simulink model "ThreeLevel_Ttype_OffGrid_Inverter_Sim"  (R2022b)
settings: Solver=FixedStepAuto  StartTime=0.0  StopTime=1  FixedStep=1e-6  RelTol=1e-3
undefined symbols (not defined in the file): L1
libraries: spsSeriesRLCBranchLib x14, spsMosfetLib x12, spsRMSLib x10, slpidlib x5, simulink x3, spsThreePhaseVIMeasurementLib x3, spsVoltageMeasurementLib x3, spsDCVoltageSourceLib x1, spsGroundLib x1, spsPower3phInstantaneousLib x1, sps_lib x1
(part 1 of 2)
settings Model: Creator=XIAO  LastModifiedBy=XIAO
settings SolverCC: AutoInsertRateTranBlk=on
settings DataIOCC: ReturnWorkspaceOutputs=off

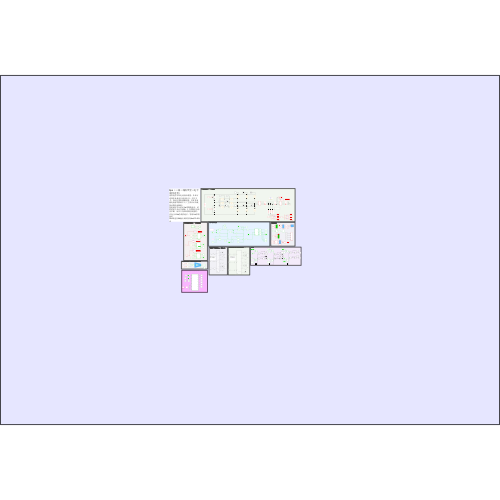
[thumbnail: Simulink's stored preview of the top-level diagram]
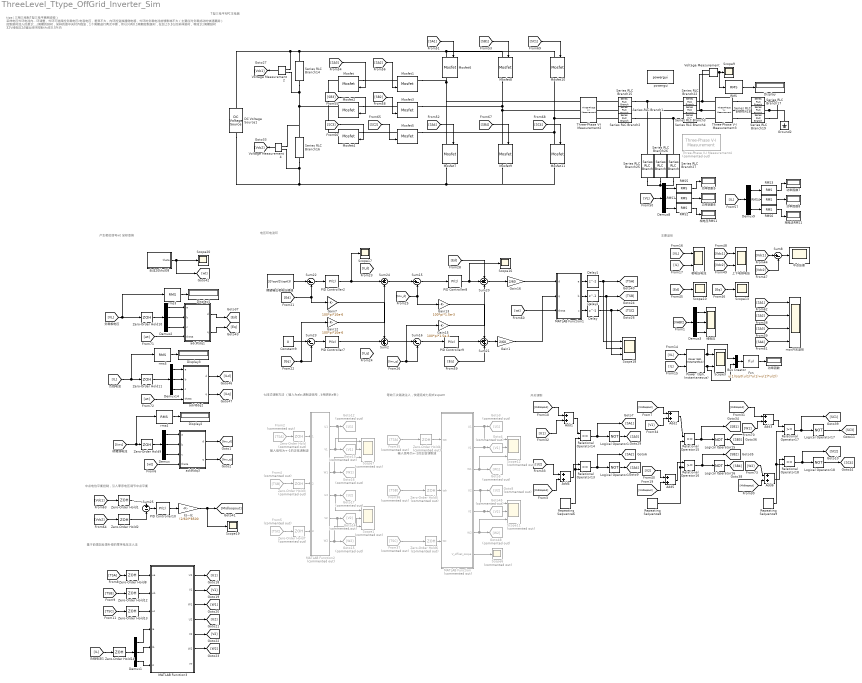
== system ThreeLevel_Ttype_OffGrid_Inverter_Sim ==
  note: 基于前馈加反馈补偿的零序电压注入法
  note: tips（三相三线制T型三电平离网逆变）
      | 采样电压外环电流内环调整，外环可选择控负载电压/电容电压，差异不大，内环控变换器侧电感，外环的负载电流前馈影响不大（主要应对负载扰动的快速跟踪）
      | 控制延时加入的是1ts周期的延时，采样的是中央对齐载波，1个周期进行两次中断，所以只有0.5周期控制延时，在加上0.5ts的采样延时，等效1ts周期延时
      | 32V线电压2A输出闭环控制thd在0.5%内
  note: T型三电平NPC主电路
  note: 主要波形
  note: 产生相位信号wt 坐标变换
  note: 电压环电流环
  note: 中点电位平衡控制，引入零序电压调节中点平衡
  note: 开关调制
  note: 输入信号为+-1的正弦调制波
  note: 等效三次谐波注入，快速完成七段式svpwm
  note: 七段式调制方法
      | （输入为abc调制波信号，b相滞后a相）
  note: 输入信号为+-1的正弦调制波
  Add{1..6} (6 alike) : Sum
  Bus Creator : BusCreator  Inputs=2
  Constant9 : Constant  Value=0
  DC Voltage Source1 : spsDCVoltageSourceLib/DC Voltage Source  Amplitude=60  Measurements=None
  Delay : Delay  DelayLength=1
  Delay1 : Delay  DelayLength=1
  Delay2 : Delay  DelayLength=1
  Demux{,1..3,8..9,14} (7 alike) : Demux  Outputs=3
  Display{,1..3} (4 alike) : Display
  Fcn : Fcn  Expr=u(1)/sqrt(u(1)*u(1)+u(2)*u(2))
  From2 : From  Commented=on  GotoTag=TSA
  From35 : From  Commented=on  GotoTag=TSA
  From36 : From  Commented=on  GotoTag=TSB
  From37 : From  Commented=on  GotoTag=TSC
  From4 : From  Commented=on  GotoTag=TSB
  From5 : From  Commented=on  GotoTag=TSC
  Gain1 : Gain  Gain=2/60
  Gain12 : Gain  Gain=100*pi*10e-6
  Gain13 : Gain  Gain=100*pi*1.5e-3
  Gain15 : Gain  Gain=100*pi*1.5e-3
  Gain16 : Gain  Gain=2/60
  Gain7 : Gain  Gain=100*pi*10e-6
  Goto12 : Goto  Commented=on  GotoTag=U1
  Goto13 : Goto  Commented=on  GotoTag=V1
  Goto14 : Goto  Commented=on  GotoTag=V2
  Goto15 : Goto  Commented=on  GotoTag=W2
  Goto16 : Goto  Commented=on  GotoTag=W1
  Goto17 : Goto  Commented=on  GotoTag=U2
  Goto3 : Goto  Commented=on  GotoTag=U1
  Goto4 : Goto  Commented=on  GotoTag=V1
  Goto45 : Goto  Commented=on  GotoTag=V2
  Goto48 : Goto  Commented=on  GotoTag=W2
  Goto5 : Goto  Commented=on  GotoTag=W1
  Goto8 : Goto  Commented=on  GotoTag=U2
  Ground2 : spsGroundLib/Ground  LConnTagsString=a
  Logical Operator{13..18} (6 alike) : Logic  Operator=NOT  AllPortsSameDT=off  OutDataTypeStr=boolean
  MATLAB Function : MATLAB Function  Commented=on  TreatAsAtomicUnit=on
  MATLAB Function1 : MATLAB Function  TreatAsAtomicUnit=on
  MATLAB Function2 : MATLAB Function  Commented=on  TreatAsAtomicUnit=on
  MATLAB Function3 : MATLAB Function  TreatAsAtomicUnit=on
  Mosfet{,1..11} (12 alike) : spsMosfetLib/Mosfet  Ron=0.1  Lon=0  Rd=0.01  Vfd=0  IC=0  Rs=1e5  Cs=inf  Measurements=on
  PID Controller10 : slpidlib/PID Controller  Controller=PI  Form=Parallel  TimeDomain=Discrete-time  UseExternalTs=off  SampleTime=-1  IntegratorMethod=Trapezoidal  FilterMethod=Forward Euler  ControllerParametersSource=internal  P=80  I=80  UseKiTs=off  D=0  N=100  UseFilter=on  TunerSelectOption=Transfer Function Based (PID Tuner App)  InitialConditionSource=internal  InitialConditionForIntegrator=0  InitialConditionForFilter=0  DifferentiatorICPrevScaledInput=0  ExternalReset=none  TrackingMode=off  Kt=1  LimitOutput=on  SatLimitsSource=internal  UpperSaturationLimit=100  LowerSaturationLimit=-100  LinearizeAsGain=on  AntiWindupMode=none  Kb=1  LimitIntegrator=off  UpperIntegratorSaturationLimit=inf  LowerIntegratorSaturationLimit=-inf  POutMin=[]  POutMax=[]  IOutMin=[]  IOutMax=[]  DOutMin=[]  DOutMax=[]  NOutMin=[]  NOutMax=[]  SumOutMin=[]  SumOutMax=[]  SaturationOutMin=[]  SaturationOutMax=[]  PParamMin=[]  PParamMax=[]  IParamMin=[]  IParamMax=[]  DParamMin=[]  DParamMax=[]  NParamMin=[]  NParamMax=[]  KbParamMin=[]  KbParamMax=[]  KtParamMin=[]  KtParamMax=[]  KbOutMin=[]  KbOutMax=[]  KtOutMin=[]  KtOutMax=[]  IntegratorOutMin=[]  IntegratorOutMax=[]  FilterOutMin=[]  FilterOutMax=[]  SumI1OutMin=[]  SumI1OutMax=[]  SumI2OutMin=[]  SumI2OutMax=[]  SumI3OutMin=[]  SumI3OutMax=[]  SumI4OutMin=[]  SumI4OutMax=[]  SumDOutMin=[]  SumDOutMax=[]  DifferentiatorOutMin=[]  DifferentiatorOutMax=[]  FilterDiffOutCoefMin=[]  FilterDiffOutCoefMax=[]  ReciprocalOutMin=[]  ReciprocalOutMax=[]  SumDenOutMin=[]  SumDenOutMax=[]  SumNumOutMin=[]  SumNumOutMax=[]  DivideOutMin=[]  DivideOutMax=[]  UdiffTsProdOutMin=[]  UdiffTsProdOutMax=[]  NTsProdOutMin=[]  NTsProdOutMax=[]  UintegralTsProdOutMin=[]  UintegralTsProdOutMax=[]  UngainTsProdOutMin=[]  UngainTsProdOutMax=[]  ClampingZeroOutDataTypeStr=Inherit: Inherit via back propagation  ClampingZeroOutMin=[]  ClampingZeroOutMax=[]  FilterDenConstantOutDataTypeStr=Inherit: Inherit via back propagation  FilterDenConstantOutMin=[]  FilterDenConstantOutMax=[]  PCopyOutDataTypeStr=Inherit: Inherit via back propagation  PCopyOutMin=[]  PCopyOutMax=[]  NCopyOutDataTypeStr=Inherit: Inherit via back propagation  NCopyOutMin=[]  NCopyOutMax=[]  IntegratorContinuousStateAttributes=''  IntegratorStateMustResolveToSignalObject=off  IntegratorRTWStateStorageClass=Auto  FilterContinuousStateAttributes=''  FilterStateMustResolveToSignalObject=off  FilterRTWStateStorageClass=Auto  ParallelPVariant=InternalParameters  IdealPVariant=Disabled  IVariant=InternalParameters  DVariant=Disabled  IntegratorVariant=Discrete  SatVariant=Enabled  AWVariant=Passthrough  PCopyVariant=Disabled  TRVariant=Disabled  FdbkBlocksVariant=Forward  IdealPFdbkVariant=Disabled  SatFdbkVariant=Disabled  DerivativeFilterVariant=Disabled  NVariant=Disabled  NCopyVariant=Disabled_SignalSpec  FilterICVariant=Disabled  IntegratorICVariant=InternalICs  ExternalResetVariant=Disabled  TRSumVariant=Passthrough  SumFdbkVariant=Disabled  SumVariant=Sum_PI  TsampFilterVariant=InternalTs  TsampNgainVariant=Passthrough  TsampIntegralVariant=Passthrough  ExternalSaturationOutDataTypeStr=Inherit: Same as second input
  PID Controller2 : slpidlib/PID Controller  Controller=PI  Form=Parallel  TimeDomain=Discrete-time  UseExternalTs=off  SampleTime=-1  IntegratorMethod=Trapezoidal  FilterMethod=Forward Euler  ControllerParametersSource=internal  P=0.04  I=53.33  UseKiTs=off  D=0  N=100  UseFilter=on  TunerSelectOption=Transfer Function Based (PID Tuner App)  InitialConditionSource=internal  InitialConditionForIntegrator=0  InitialConditionForFilter=0  DifferentiatorICPrevScaledInput=0  ExternalReset=none  TrackingMode=off  Kt=1  LimitOutput=off  SatLimitsSource=internal  UpperSaturationLimit=inf  LowerSaturationLimit=-inf  LinearizeAsGain=on  AntiWindupMode=none  Kb=1  LimitIntegrator=off  UpperIntegratorSaturationLimit=inf  LowerIntegratorSaturationLimit=-inf  POutMin=[]  POutMax=[]  IOutMin=[]  IOutMax=[]  DOutMin=[]  DOutMax=[]  NOutMin=[]  NOutMax=[]  SumOutMin=[]  SumOutMax=[]  SaturationOutMin=[]  SaturationOutMax=[]  PParamMin=[]  PParamMax=[]  IParamMin=[]  IParamMax=[]  DParamMin=[]  DParamMax=[]  NParamMin=[]  NParamMax=[]  KbParamMin=[]  KbParamMax=[]  KtParamMin=[]  KtParamMax=[]  KbOutMin=[]  KbOutMax=[]  KtOutMin=[]  KtOutMax=[]  IntegratorOutMin=[]  IntegratorOutMax=[]  FilterOutMin=[]  FilterOutMax=[]  SumI1OutMin=[]  SumI1OutMax=[]  SumI2OutMin=[]  SumI2OutMax=[]  SumI3OutMin=[]  SumI3OutMax=[]  SumI4OutMin=[]  SumI4OutMax=[]  SumDOutMin=[]  SumDOutMax=[]  DifferentiatorOutMin=[]  DifferentiatorOutMax=[]  FilterDiffOutCoefMin=[]  FilterDiffOutCoefMax=[]  ReciprocalOutMin=[]  ReciprocalOutMax=[]  SumDenOutMin=[]  SumDenOutMax=[]  SumNumOutMin=[]  SumNumOutMax=[]  DivideOutMin=[]  DivideOutMax=[]  UdiffTsProdOutMin=[]  UdiffTsProdOutMax=[]  NTsProdOutMin=[]  NTsProdOutMax=[]  UintegralTsProdOutMin=[]  UintegralTsProdOutMax=[]  UngainTsProdOutMin=[]  UngainTsProdOutMax=[]  ClampingZeroOutDataTypeStr=Inherit: Inherit via back propagation  ClampingZeroOutMin=[]  ClampingZeroOutMax=[]  FilterDenConstantOutDataTypeStr=Inherit: Inherit via back propagation  FilterDenConstantOutMin=[]  FilterDenConstantOutMax=[]  PCopyOutDataTypeStr=Inherit: Inherit via back propagation  PCopyOutMin=[]  PCopyOutMax=[]  NCopyOutDataTypeStr=Inherit: Inherit via back propagation  NCopyOutMin=[]  NCopyOutMax=[]  IntegratorContinuousStateAttributes=''  IntegratorStateMustResolveToSignalObject=off  IntegratorRTWStateStorageClass=Auto  FilterContinuousStateAttributes=''  FilterStateMustResolveToSignalObject=off  FilterRTWStateStorageClass=Auto  ParallelPVariant=InternalParameters  IdealPVariant=Disabled  IVariant=InternalParameters  DVariant=Disabled  IntegratorVariant=Discrete  SatVariant=Disabled  AWVariant=Passthrough  PCopyVariant=Disabled  TRVariant=Disabled  FdbkBlocksVariant=Forward  IdealPFdbkVariant=Disabled  SatFdbkVariant=Disabled  DerivativeFilterVariant=Disabled  NVariant=Disabled  NCopyVariant=Disabled_SignalSpec  FilterICVariant=Disabled  IntegratorICVariant=InternalICs  ExternalResetVariant=Disabled  TRSumVariant=Passthrough  SumFdbkVariant=Disabled  SumVariant=Sum_PI  TsampFilterVariant=InternalTs  TsampNgainVariant=Passthrough  TsampIntegralVariant=Passthrough  ExternalSaturationOutDataTypeStr=Inherit: Same as second input
  PID Controller7 : slpidlib/PID Controller  Controller=PI  Form=Parallel  TimeDomain=Discrete-time  UseExternalTs=off  SampleTime=-1  IntegratorMethod=Trapezoidal  FilterMethod=Forward Euler  ControllerParametersSource=internal  P=0.04  I=53.33  UseKiTs=off  D=0  N=100  UseFilter=on  TunerSelectOption=Transfer Function Based (PID Tuner App)  InitialConditionSource=internal  InitialConditionForIntegrator=0  InitialConditionForFilter=0  DifferentiatorICPrevScaledInput=0  ExternalReset=none  TrackingMode=off  Kt=1  LimitOutput=off  SatLimitsSource=internal  UpperSaturationLimit=inf  LowerSaturationLimit=-inf  LinearizeAsGain=on  AntiWindupMode=none  Kb=1  LimitIntegrator=off  UpperIntegratorSaturationLimit=inf  LowerIntegratorSaturationLimit=-inf  POutMin=[]  POutMax=[]  IOutMin=[]  IOutMax=[]  DOutMin=[]  DOutMax=[]  NOutMin=[]  NOutMax=[]  SumOutMin=[]  SumOutMax=[]  SaturationOutMin=[]  SaturationOutMax=[]  PParamMin=[]  PParamMax=[]  IParamMin=[]  IParamMax=[]  DParamMin=[]  DParamMax=[]  NParamMin=[]  NParamMax=[]  KbParamMin=[]  KbParamMax=[]  KtParamMin=[]  KtParamMax=[]  KbOutMin=[]  KbOutMax=[]  KtOutMin=[]  KtOutMax=[]  IntegratorOutMin=[]  IntegratorOutMax=[]  FilterOutMin=[]  FilterOutMax=[]  SumI1OutMin=[]  SumI1OutMax=[]  SumI2OutMin=[]  SumI2OutMax=[]  SumI3OutMin=[]  SumI3OutMax=[]  SumI4OutMin=[]  SumI4OutMax=[]  SumDOutMin=[]  SumDOutMax=[]  DifferentiatorOutMin=[]  DifferentiatorOutMax=[]  FilterDiffOutCoefMin=[]  FilterDiffOutCoefMax=[]  ReciprocalOutMin=[]  ReciprocalOutMax=[]  SumDenOutMin=[]  SumDenOutMax=[]  SumNumOutMin=[]  SumNumOutMax=[]  DivideOutMin=[]  DivideOutMax=[]  UdiffTsProdOutMin=[]  UdiffTsProdOutMax=[]  NTsProdOutMin=[]  NTsProdOutMax=[]  UintegralTsProdOutMin=[]  UintegralTsProdOutMax=[]  UngainTsProdOutMin=[]  UngainTsProdOutMax=[]  ClampingZeroOutDataTypeStr=Inherit: Inherit via back propagation  ClampingZeroOutMin=[]  ClampingZeroOutMax=[]  FilterDenConstantOutDataTypeStr=Inherit: Inherit via back propagation  FilterDenConstantOutMin=[]  FilterDenConstantOutMax=[]  PCopyOutDataTypeStr=Inherit: Inherit via back propagation  PCopyOutMin=[]  PCopyOutMax=[]  NCopyOutDataTypeStr=Inherit: Inherit via back propagation  NCopyOutMin=[]  NCopyOutMax=[]  IntegratorContinuousStateAttributes=''  IntegratorStateMustResolveToSignalObject=off  IntegratorRTWStateStorageClass=Auto  FilterContinuousStateAttributes=''  FilterStateMustResolveToSignalObject=off  FilterRTWStateStorageClass=Auto  ParallelPVariant=InternalParameters  IdealPVariant=Disabled  IVariant=InternalParameters  DVariant=Disabled  IntegratorVariant=Discrete  SatVariant=Disabled  AWVariant=Passthrough  PCopyVariant=Disabled  TRVariant=Disabled  FdbkBlocksVariant=Forward  IdealPFdbkVariant=Disabled  SatFdbkVariant=Disabled  DerivativeFilterVariant=Disabled  NVariant=Disabled  NCopyVariant=Disabled_SignalSpec  FilterICVariant=Disabled  IntegratorICVariant=InternalICs  ExternalResetVariant=Disabled  TRSumVariant=Passthrough  SumFdbkVariant=Disabled  SumVariant=Sum_PI  TsampFilterVariant=InternalTs  TsampNgainVariant=Passthrough  TsampIntegralVariant=Passthrough  ExternalSaturationOutDataTypeStr=Inherit: Same as second input
  PID Controller8 : slpidlib/PID Controller  Controller=PI  Form=Parallel  TimeDomain=Discrete-time  UseExternalTs=off  SampleTime=-1  IntegratorMethod=Trapezoidal  FilterMethod=Forward Euler  ControllerParametersSource=internal  P=10  I=233  UseKiTs=off  D=0  N=100  UseFilter=on  TunerSelectOption=Transfer Function Based (PID Tuner App)  InitialConditionSource=internal  InitialConditionForIntegrator=0  InitialConditionForFilter=0  DifferentiatorICPrevScaledInput=0  ExternalReset=none  TrackingMode=off  Kt=1  LimitOutput=off  SatLimitsSource=internal  UpperSaturationLimit=inf  LowerSaturationLimit=-inf  LinearizeAsGain=on  AntiWindupMode=none  Kb=1  LimitIntegrator=off  UpperIntegratorSaturationLimit=inf  LowerIntegratorSaturationLimit=-inf  POutMin=[]  POutMax=[]  IOutMin=[]  IOutMax=[]  DOutMin=[]  DOutMax=[]  NOutMin=[]  NOutMax=[]  SumOutMin=[]  SumOutMax=[]  SaturationOutMin=[]  SaturationOutMax=[]  PParamMin=[]  PParamMax=[]  IParamMin=[]  IParamMax=[]  DParamMin=[]  DParamMax=[]  NParamMin=[]  NParamMax=[]  KbParamMin=[]  KbParamMax=[]  KtParamMin=[]  KtParamMax=[]  KbOutMin=[]  KbOutMax=[]  KtOutMin=[]  KtOutMax=[]  IntegratorOutMin=[]  IntegratorOutMax=[]  FilterOutMin=[]  FilterOutMax=[]  SumI1OutMin=[]  SumI1OutMax=[]  SumI2OutMin=[]  SumI2OutMax=[]  SumI3OutMin=[]  SumI3OutMax=[]  SumI4OutMin=[]  SumI4OutMax=[]  SumDOutMin=[]  SumDOutMax=[]  DifferentiatorOutMin=[]  DifferentiatorOutMax=[]  FilterDiffOutCoefMin=[]  FilterDiffOutCoefMax=[]  ReciprocalOutMin=[]  ReciprocalOutMax=[]  SumDenOutMin=[]  SumDenOutMax=[]  SumNumOutMin=[]  SumNumOutMax=[]  DivideOutMin=[]  DivideOutMax=[]  UdiffTsProdOutMin=[]  UdiffTsProdOutMax=[]  NTsProdOutMin=[]  NTsProdOutMax=[]  UintegralTsProdOutMin=[]  UintegralTsProdOutMax=[]  UngainTsProdOutMin=[]  UngainTsProdOutMax=[]  ClampingZeroOutDataTypeStr=Inherit: Inherit via back propagation  ClampingZeroOutMin=[]  ClampingZeroOutMax=[]  FilterDenConstantOutDataTypeStr=Inherit: Inherit via back propagation  FilterDenConstantOutMin=[]  FilterDenConstantOutMax=[]  PCopyOutDataTypeStr=Inherit: Inherit via back propagation  PCopyOutMin=[]  PCopyOutMax=[]  NCopyOutDataTypeStr=Inherit: Inherit via back propagation  NCopyOutMin=[]  NCopyOutMax=[]  IntegratorContinuousStateAttributes=''  IntegratorStateMustResolveToSignalObject=off  IntegratorRTWStateStorageClass=Auto  FilterContinuousStateAttributes=''  FilterStateMustResolveToSignalObject=off  FilterRTWStateStorageClass=Auto  ParallelPVariant=InternalParameters  IdealPVariant=Disabled  IVariant=InternalParameters  DVariant=Disabled  IntegratorVariant=Discrete  SatVariant=Disabled  AWVariant=Passthrough  PCopyVariant=Disabled  TRVariant=Disabled  FdbkBlocksVariant=Forward  IdealPFdbkVariant=Disabled  SatFdbkVariant=Disabled  DerivativeFilterVariant=Disabled  NVariant=Disabled  NCopyVariant=Disabled_SignalSpec  FilterICVariant=Disabled  IntegratorICVariant=InternalICs  ExternalResetVariant=Disabled  TRSumVariant=Passthrough  SumFdbkVariant=Disabled  SumVariant=Sum_PI  TsampFilterVariant=InternalTs  TsampNgainVariant=Passthrough  TsampIntegralVariant=Passthrough  ExternalSaturationOutDataTypeStr=Inherit: Same as second input
  PID Controller9 : slpidlib/PID Controller  Controller=PI  Form=Parallel  TimeDomain=Discrete-time  UseExternalTs=off  SampleTime=-1  IntegratorMethod=Trapezoidal  FilterMethod=Forward Euler  ControllerParametersSource=internal  P=10  I=233  UseKiTs=off  D=0  N=100  UseFilter=on  TunerSelectOption=Transfer Function Based (PID Tuner App)  InitialConditionSource=internal  InitialConditionForIntegrator=0  InitialConditionForFilter=0  DifferentiatorICPrevScaledInput=0  ExternalReset=none  TrackingMode=off  Kt=1  LimitOutput=off  SatLimitsSource=internal  UpperSaturationLimit=inf  LowerSaturationLimit=-inf  LinearizeAsGain=on  AntiWindupMode=none  Kb=1  LimitIntegrator=off  UpperIntegratorSaturationLimit=inf  LowerIntegratorSaturationLimit=-inf  POutMin=[]  POutMax=[]  IOutMin=[]  IOutMax=[]  DOutMin=[]  DOutMax=[]  NOutMin=[]  NOutMax=[]  SumOutMin=[]  SumOutMax=[]  SaturationOutMin=[]  SaturationOutMax=[]  PParamMin=[]  PParamMax=[]  IParamMin=[]  IParamMax=[]  DParamMin=[]  DParamMax=[]  NParamMin=[]  NParamMax=[]  KbParamMin=[]  KbParamMax=[]  KtParamMin=[]  KtParamMax=[]  KbOutMin=[]  KbOutMax=[]  KtOutMin=[]  KtOutMax=[]  IntegratorOutMin=[]  IntegratorOutMax=[]  FilterOutMin=[]  FilterOutMax=[]  SumI1OutMin=[]  SumI1OutMax=[]  SumI2OutMin=[]  SumI2OutMax=[]  SumI3OutMin=[]  SumI3OutMax=[]  SumI4OutMin=[]  SumI4OutMax=[]  SumDOutMin=[]  SumDOutMax=[]  DifferentiatorOutMin=[]  DifferentiatorOutMax=[]  FilterDiffOutCoefMin=[]  FilterDiffOutCoefMax=[]  ReciprocalOutMin=[]  ReciprocalOutMax=[]  SumDenOutMin=[]  SumDenOutMax=[]  SumNumOutMin=[]  SumNumOutMax=[]  DivideOutMin=[]  DivideOutMax=[]  UdiffTsProdOutMin=[]  UdiffTsProdOutMax=[]  NTsProdOutMin=[]  NTsProdOutMax=[]  UintegralTsProdOutMin=[]  UintegralTsProdOutMax=[]  UngainTsProdOutMin=[]  UngainTsProdOutMax=[]  ClampingZeroOutDataTypeStr=Inherit: Inherit via back propagation  ClampingZeroOutMin=[]  ClampingZeroOutMax=[]  FilterDenConstantOutDataTypeStr=Inherit: Inherit via back propagation  FilterDenConstantOutMin=[]  FilterDenConstantOutMax=[]  PCopyOutDataTypeStr=Inherit: Inherit via back propagation  PCopyOutMin=[]  PCopyOutMax=[]  NCopyOutDataTypeStr=Inherit: Inherit via back propagation  NCopyOutMin=[]  NCopyOutMax=[]  IntegratorContinuousStateAttributes=''  IntegratorStateMustResolveToSignalObject=off  IntegratorRTWStateStorageClass=Auto  FilterContinuousStateAttributes=''  FilterStateMustResolveToSignalObject=off  FilterRTWStateStorageClass=Auto  ParallelPVariant=InternalParameters  IdealPVariant=Disabled  IVariant=InternalParameters  DVariant=Disabled  IntegratorVariant=Discrete  SatVariant=Disabled  AWVariant=Passthrough  PCopyVariant=Disabled  TRVariant=Disabled  FdbkBlocksVariant=Forward  IdealPFdbkVariant=Disabled  SatFdbkVariant=Disabled  DerivativeFilterVariant=Disabled  NVariant=Disabled  NCopyVariant=Disabled_SignalSpec  FilterICVariant=Disabled  IntegratorICVariant=InternalICs  ExternalResetVariant=Disabled  TRSumVariant=Passthrough  SumFdbkVariant=Disabled  SumVariant=Sum_PI  TsampFilterVariant=InternalTs  TsampNgainVariant=Passthrough  TsampIntegralVariant=Passthrough  ExternalSaturationOutDataTypeStr=Inherit: Same as second input
  "Power (3ph, Instantaneous)" : spsPower3phInstantaneousLib/Power (3ph, Instantaneous)
  RMS : spsRMSLib/RMS  TrueRMS=on  Freq=50  RMSInit=120  Ts=1e-6
  RMS{1..6} (6 alike) : spsRMSLib/RMS  TrueRMS=on  Freq=50  RMSInit=0  Ts=1e-6
  Relational Operator{13..18} (6 alike) : RelationalOperator  OutDataTypeStr=boolean  RndMeth=Simplest  InputSameDT=off
  Repeating Sequence6 : simulink/Sources/Repeating Sequence  rep_seq_t="[0  5e-5  1e-4]"  rep_seq_y=[0 8500 0]
  Repeating Sequence8 : simulink/Sources/Repeating Sequence  rep_seq_t="[0  5e-5  1e-4]"  rep_seq_y=[0 8500 0]
  Repeating Sequence9 : simulink/Sources/Repeating Sequence  rep_seq_t="[0  5e-5  1e-4]"  rep_seq_y=[0 8500 0]
  Scope{1,7,11..12} (4 alike) : Scope  Commented=on  NumInputPorts=3
  Scope{9..10,13,16..17,19..20} (7 alike) : Scope
  Scope18 : Scope  NumInputPorts=3
  Scope3 : Scope  NumInputPorts=2
  Scope6 : Scope  Commented=on
  Series RLC Branch1 : spsSeriesRLCBranchLib/Series RLC Branch  LConnTagsString=__new0  RConnTagsString=__new0  BranchType=RL  Resistance=4e-3  Inductance=1.5e-3  SetiL0=off  InitialCurrent=0  Capacitance=5.6e-3  Setx0=off  InitialVoltage=0  Measurements=None
  Series RLC Branch14 : spsSeriesRLCBranchLib/Series RLC Branch  LConnTagsString=__new0  RConnTagsString=__new0  BranchType=RC  Resistance=0.001  Inductance=1e-3  SetiL0=off  InitialCurrent=0  Capacitance=1000e-6  Setx0=off  InitialVoltage=260  Measurements=None
  Series RLC Branch15 : spsSeriesRLCBranchLib/Series RLC Branch  LConnTagsString=__new0  RConnTagsString=__new0  BranchType=RL  Resistance=4e-3  Inductance=1.5e-3  SetiL0=off  InitialCurrent=0  Capacitance=5.6e-3  Setx0=off  InitialVoltage=0  Measurements=None
  Series RLC Branch16 : spsSeriesRLCBranchLib/Series RLC Branch  LConnTagsString=__new0  RConnTagsString=__new0  BranchType=RC  Resistance=0.001  Inductance=1e-3  SetiL0=off  InitialCurrent=0  Capacitance=1000e-6  Setx0=off  InitialVoltage=200  Measurements=None
  Series RLC Branch17 : spsSeriesRLCBranchLib/Series RLC Branch  LConnTagsString=__new0  RConnTagsString=__new0  BranchType=RLC  Resistance=9.24  Inductance=0  SetiL0=off  InitialCurrent=0  Capacitance=0  Setx0=off  InitialVoltage=0  Measurements=None
  Series RLC Branch18 : spsSeriesRLCBranchLib/Series RLC Branch  LConnTagsString=__new0  RConnTagsString=__new0  BranchType=RLC  Resistance=9.24  Inductance=0  SetiL0=off  InitialCurrent=0  Capacitance=0  Setx0=off  InitialVoltage=0  Measurements=None
  Series RLC Branch19 : spsSeriesRLCBranchLib/Series RLC Branch  LConnTagsString=__new0  RConnTagsString=__new0  BranchType=RLC  Resistance=9.24  Inductance=0  SetiL0=off  InitialCurrent=0  Capacitance=0  Setx0=off  InitialVoltage=0  Measurements=None
  Series RLC Branch2 : spsSeriesRLCBranchLib/Series RLC Branch  LConnTagsString=__new0  RConnTagsString=__new0  BranchType=RL  Resistance=4e-3  Inductance=1.5e-3  SetiL0=off  InitialCurrent=0  Capacitance=5.6e-3  Setx0=off  InitialVoltage=0  Measurements=None
  Series RLC Branch22 : spsSeriesRLCBranchLib/Series RLC Branch  LConnTagsString=__new0  RConnTagsString=__new0  BranchType=L  Resistance=1e-6  Inductance=330e-6  SetiL0=off  InitialCurrent=0  Capacitance=5.6e-3  Setx0=off  InitialVoltage=0  Measurements=None
  Series RLC Branch25 : spsSeriesRLCBranchLib/Series RLC Branch  LConnTagsString=__new0  RConnTagsString=__new0  BranchType=RC  Resistance=1.5  Inductance=L1  SetiL0=off  InitialCurrent=0  Capacitance=10e-6  Setx0=off  InitialVoltage=0  Measurements=None
  Series RLC Branch26 : spsSeriesRLCBranchLib/Series RLC Branch  LConnTagsString=__new0  RConnTagsString=__new0  BranchType=RC  Resistance=1.5  Inductance=L1  SetiL0=off  InitialCurrent=0  Capacitance=10e-6  Setx0=off  InitialVoltage=0  Measurements=None
  Series RLC Branch27 : spsSeriesRLCBranchLib/Series RLC Branch  LConnTagsString=__new0  RConnTagsString=__new0  BranchType=RC  Resistance=1.5  Inductance=L1  SetiL0=off  InitialCurrent=0  Capacitance=10.0e-6  Setx0=off  InitialVoltage=0  Measurements=None
  Series RLC Branch3 : spsSeriesRLCBranchLib/Series RLC Branch  LConnTagsString=__new0  RConnTagsString=__new0  BranchType=L  Resistance=1e-6  Inductance=330e-6  SetiL0=off  InitialCurrent=0  Capacitance=5.6e-3  Setx0=off  InitialVoltage=0  Measurements=None
  Series RLC Branch4 : spsSeriesRLCBranchLib/Series RLC Branch  LConnTagsString=__new0  RConnTagsString=__new0  BranchType=L  Resistance=1e-6  Inductance=330e-6  SetiL0=off  InitialCurrent=0  Capacitance=5.6e-3  Setx0=off  InitialVoltage=0  Measurements=None
  Sum{8,15..16,22..23} (5 alike) : Sum  Inputs=|+-
  Sum2 : Sum  Inputs=+++
  Sum20 : Sum  Inputs=++-
  Sum21 : Sum  Inputs=+++
  Sum24 : Sum  Inputs=++-
  Sum25 : Sum  Inputs=+-
  Three-Phase V-I Measurement2 : spsThreePhaseVIMeasurementLib/Three-Phase V-I Measurement  VoltageMeasurement=phase-to-phase  SetLabelV=on  LabelV=VABC  Vpu=off  VpuLL=off  CurrentMeasurement=yes  SetLabelI=on  LabelI=Iinv  Ipu=off  Pbase=100e6  Vbase=500e3  OutputType=Complex  PhasorSimulation=off  PSBequivalent=0
  Three-Phase V-I Measurement3 : spsThreePhaseVIMeasurementLib/Three-Phase V-I Measurement  VoltageMeasurement=phase-to-ground  SetLabelV=on  LabelV=VL  Vpu=off  VpuLL=off  CurrentMeasurement=yes  SetLabelI=on  LabelI=IL  Ipu=off  Pbase=100e6  Vbase=500e3  OutputType=Complex  PhasorSimulation=off  PSBequivalent=0
  Three-Phase V-I Measurement4 : spsThreePhaseVIMeasurementLib/Three-Phase V-I Measurement  Commented=on  VoltageMeasurement=phase-to-ground  SetLabelV=on  LabelV=VL  Vpu=off  VpuLL=off  CurrentMeasurement=yes  SetLabelI=on  LabelI=IL  Ipu=off  Pbase=100e6  Vbase=500e3  OutputType=Complex  PhasorSimulation=off  PSBequivalent=0
  Voltage Measurement : spsVoltageMeasurementLib/Voltage Measurement  PhasorSimulation=off  OutputType=Complex  PSBequivalent=0
  Voltage Measurement2 : spsVoltageMeasurementLib/Voltage Measurement  PhasorSimulation=off  OutputType=Complex  PSBequivalent=0
  Voltage Measurement4 : spsVoltageMeasurementLib/Voltage Measurement  PhasorSimulation=off  OutputType=Complex  PSBequivalent=0
  Zero-Order Hold{,3..7} (6 alike) : ZeroOrderHold  Commented=on  SampleTime=5e-5
  Zero-Order Hold{1..2,8..14} (9 alike) : ZeroOrderHold  SampleTime=5e-5
  adc转dq1 : MATLAB Function  TreatAsAtomicUnit=on
  adc转dq2 : MATLAB Function  TreatAsAtomicUnit=on
  adc转dq3 : MATLAB Function  TreatAsAtomicUnit=on
  mos开关波形 : Scope  NumInputPorts=4
  powergui : sps_lib/powergui  Priority=1  SimulationMode=Discrete  SampleTime=1e-6  frequency=60  Iterations=50  frequencyindice=0  Pbase=100e6  ErrMax=1e-4  UnitsV=kV  UnitsW=MW  buscounter=0  FunctionMessages=off  echomessages=off  EnableUseOfTLC=off  CurrentSourceSwitches=off  DisableSnubberDevices=off  DisableRonSwitches=off  DisableVfSwitches=off  DisplayEquations=off  AutomaticDiscreteSolvers=off  SolverType=Tustin/Backward Euler (TBE)  Interpol=off  ExternalGateDelay=off  methode=off  Ts=100  x0status=blocks  SPID=on  SwTol=0  HookPort=off  NonlinearTolerance=1e-4  nMaxIteration=100  ContinueOnMaxIteration=off  RestoreLinks=warning  ResistiveCurrentMeasurement=off  Frange=[0:2:500]  Ylog=off  Xlog=on  ShowGrid=off  save=off  variable=ZData  structure=0  ZoomFFT=off  StartTime=0.0  cycles=1  DisplayStyle=1  fundamental=60  FreqAxis=off  MaxFrequency=1000  frequencyindicesteady=1  RmsSteady=1  display=off
  rms3 : spsRMSLib/RMS  TrueRMS=on  Freq=50  RMSInit=120  Ts=1e-6
  rms4 : spsRMSLib/RMS  TrueRMS=on  Freq=50  RMSInit=120  Ts=1e-6
  rms5 : spsRMSLib/RMS  TrueRMS=on  Freq=50  RMSInit=120  Ts=1e-6
  上下电容电压 : Scope  NumInputPorts=2
  中点压差 : Scope
  功率因数{,5..8} (5 alike) : Display
  归一化 : Gain  Gain=(2/60)*8500
  期望输出相电压峰值 : Constant  Value=32*sqrt(2)/sqrt(3)
  生成20khz的θ : MATLAB Function  TreatAsAtomicUnit=on  SystemSampleTime=5e-5
  相电压RMS1 : Display
  相电压电流 : Scope  NumInputPorts=2
  相电流RMS1 : Display
  线电压 : Scope  NumInputPorts=3
  wires:
  [VL] -> 相电压电流/1
  [VL] -> "Power (3ph, Instantaneous)"/1
  Fcn/1 -> 功率因数/1
  [Vdc1] -> 上下电容电压/1
  RMS/1 -> Display/1
  Demux9/2 -> RMS4/1
  Voltage Measurement/1 -> RMS/1, Scope9/1
  [Vdc2] -> Sum8/2
  "Power (3ph, Instantaneous)"/2 -> Bus Creator/2, Scope3/2
  [Vdc1] -> Sum8/1
  RMS6/1 -> 相电流RMS1/1
  Bus Creator/1 -> Fcn/1
  [VABC] -> Demux3/1
  [IL] -> "Power (3ph, Instantaneous)"/2
  Demux3/2 -> 线电压/2
  RMS3/1 -> 功率因数7/1
  "Power (3ph, Instantaneous)"/1 -> Bus Creator/1, Scope3/1
  [Ed] -> Scope10/1
  RMS4/1 -> 功率因数8/1
  Demux9/3 -> RMS6/1
  Demux9/1 -> RMS3/1
  RMS5/1 -> 功率因数5/1
  RMS1/1 -> 功率因数6/1
  Demux3/3 -> 线电压/3
  Demux8/3 -> RMS2/1
  [IL] -> 相电压电流/2
  RMS2/1 -> 相电压RMS1/1
  Demux8/1 -> RMS5/1
  Demux8/2 -> RMS1/1
  Demux3/1 -> 线电压/1
  [Vdc2] -> 上下电容电压/2
  [VL] -> Demux8/1
  [IL] -> Demux9/1
  [Eq] -> Scope13/1
  Sum8/1 -> 中点压差/1
  [SA3] -> Mosfet/1
  Voltage Measurement4/1 -> [Vdc2]
  [SB4] -> Mosfet9/1
  [SB3] -> Mosfet2/1
  [SB2] -> Mosfet3/1
  [SC3] -> Mosfet4/1
  [SC2] -> Mosfet5/1
  [SB1] -> Mosfet8/1
  [SC1] -> Mosfet10/1
  Voltage Measurement2/1 -> [Vdc1]
  [SA4] -> Mosfet7/1
  [SC4] -> Mosfet11/1
  [SA1] -> Mosfet6/1
  [SA2] -> Mosfet1/1
  [Ed] -> Gain7/1, Sum22/2
  Gain7/1 -> Sum2/1
  PID Controller2/1 -> Scope17/1, Sum24/2
  Sum22/1 -> PID Controller2/1
  Gain15/1 -> Sum20/3
  MATLAB Function1/3(c) -> Delay/1
  Sum24/1 -> Sum15/1
  期望输出相电压峰值/1 -> Sum22/1
  PID Controller7/1 -> Sum2/2
  Sum2/1 -> Sum16/1
  Sum15/1 -> PID Controller8/1
  Gain12/1 -> Sum24/3
  Sum16/1 -> PID Controller9/1
  [Iinv_q] -> Gain15/1, Sum16/2
  Gain13/1 -> Sum21/1
  PID Controller9/1 -> Sum21/2
  Sum23/1 -> PID Controller7/1
  [Ed] -> Sum20/1
  Sum21/1 -> Gain1/1
  PID Controller8/1 -> Scope16/1, Sum20/2
  [Iinv_d] -> Gain13/1, Sum15/2
  Sum20/1 -> Gain16/1
  MATLAB Function1/1(a) -> Delay1/1
  Constant9/1 -> Sum23/1
  MATLAB Function1/2(b) -> Delay2/1
  Gain1/1 -> MATLAB Function1/2(q)
  [Eq] -> Gain12/1, Sum23/2
  [Eq] -> Sum21/3
  [Vdc2] -> Zero-Order Hold2/1
  PID Controller10/1 -> 归一化/1
  [Vdc1] -> Zero-Order Hold1/1
  归一化/1 -> [Midloopout], Scope19/1
  Sum25/1 -> PID Controller10/1
  Zero-Order Hold1/1 -> Sum25/1
  Zero-Order Hold2/1 -> Sum25/2
  生成20khz的θ/1(theta) -> Scope20/1, [wt]
  rms3/1 -> Display1/1
  Zero-Order Hold11/1 -> Demux14/1
  [wt] -> adc转dq1/4(theta)
  Demux14/1 -> adc转dq2/1(a)
  Demux14/3 -> adc转dq2/3(c)
  [IL] -> rms5/1, Zero-Order Hold11/1
  rms5/1 -> Display3/1
  adc转dq2/1(d) -> [ILd]
  adc转dq2/2(q) -> [ILq]
  [VL] -> rms3/1, Zero-Order Hold10/1
  Zero-Order Hold10/1 -> Demux2/1
  Demux2/1 -> adc转dq1/1(a)
  Demux2/2 -> adc转dq1/2(b)
  Demux2/3 -> adc转dq1/3(c)
  adc转dq1/2(q) -> [Eq]
  adc转dq1/1(d) -> [Ed]
  Demux14/2 -> adc转dq2/2(b)
  [wt] -> adc转dq2/4(theta)
  Demux/3 -> adc转dq3/3(c)
  Zero-Order Hold9/1 -> Demux/1
  [Iinv] -> rms4/1, Zero-Order Hold9/1
  rms4/1 -> Display2/1
  adc转dq3/2(q) -> [Iinv_q]
  adc转dq3/1(d) -> [Iinv_d]
  Demux/1 -> adc转dq3/1(a)
  Demux/2 -> adc转dq3/2(b)
  [wt] -> adc转dq3/4(theta)
  Add4/1 -> Relational Operator13/1
  MATLAB Function/1(U1) -> Scope12/1, Goto3/1
  [SA2] -> mos开关波形/2
  [Midloopout] -> Add3/1
  Add2/1 -> Relational Operator15/1
  [SA3] -> mos开关波形/3
  [W1] -> Add3/2
  [Midloopout] -> Add4/2
  Relational Operator13/1 -> [SA2], Logical Operator14/1
  Logical Operator18/1 -> [SC4]
  MATLAB Function/3(W1) -> Scope12/3, Goto5/1
  [SA4] -> mos开关波形/4
  MATLAB Function/5(V2) -> Scope11/2, Goto45/1
  MATLAB Function/6(W2) -> Scope11/3, Goto48/1
  [U2] -> Add4/1
  Relational Operator16/1 -> Logical Operator16/1, [SB2]
  [Midloopout] -> Add6/2
  Relational Operator17/1 -> [SC1], Logical Operator17/1
  Logical Operator17/1 -> [SC3]
  Zero-Order Hold4/1 -> MATLAB Function/1(tsa)
  Logical Operator15/1 -> [SB3]
  MATLAB Function/7(V_offset_scope) -> Scope6/1
  MATLAB Function/2(V1) -> Scope12/2, Goto4/1
  Logical Operator13/1 -> [SA3]
  Add5/1 -> Relational Operator16/1
  [Midloopout] -> Add1/1
  [Midloopout] -> Add2/1
  Relational Operator14/1 -> [SA1], Logical Operator13/1
  From35/1 -> Zero-Order Hold4/1
  From36/1 -> Zero-Order Hold5/1
  Logical Operator16/1 -> [SB4]
  Add3/1 -> Relational Operator17/1
  Repeating Sequence6/1 -> Relational Operator14/2, Relational Operator13/2
  Relational Operator15/1 -> Logical Operator15/1, [SB1]
  [U1] -> Add1/2
  Repeating Sequence9/1 -> Relational Operator18/2, Relational Operator17/2
  [SA1] -> mos开关波形/1
  Zero-Order Hold5/1 -> MATLAB Function/2(tsb)
  Logical Operator14/1 -> [SA4]
  MATLAB Function/4(U2) -> Scope11/1, Goto8/1
  [V1] -> Add2/2
  [V2] -> Add5/1
  From37/1 -> Zero-Order Hold6/1
  Relational Operator18/1 -> [SC2], Logical Operator18/1
  [Midloopout] -> Add5/2
  Add1/1 -> Relational Operator14/1
  Add6/1 -> Relational Operator18/1
  Zero-Order Hold6/1 -> MATLAB Function/3(tsc)
  Repeating Sequence8/1 -> Relational Operator15/2, Relational Operator16/2
  [W2] -> Add6/1
  [wt] -> MATLAB Function1/3(theta)
  Zero-Order Hold/1 -> MATLAB Function2/1(Ua_norm)
  Zero-Order Hold7/1 -> MATLAB Function2/3(Uc_norm)
  Zero-Order Hold3/1 -> MATLAB Function2/2(Ub_norm)
  MATLAB Function2/6(W2) -> Scope1/3, Goto15/1
  MATLAB Function2/5(V2) -> Scope1/2, Goto14/1
  MATLAB Function2/4(U2) -> Scope1/1, Goto17/1
  MATLAB Function2/3(W1) -> Scope7/3, Goto16/1
  MATLAB Function2/2(V1) -> Scope7/2, Goto13/1
  MATLAB Function2/1(U1) -> Scope7/1, Goto12/1
  From2/1 -> Zero-Order Hold/1
  From4/1 -> Zero-Order Hold3/1
  From5/1 -> Zero-Order Hold7/1
  Gain16/1 -> MATLAB Function1/1(d)
  Delay1/1 -> Scope18/1, [TSA]
  Delay2/1 -> Scope18/2, [TSB]
  Delay/1 -> [TSC], Scope18/3
  [TSA] -> Zero-Order Hold8/1
  [TSB] -> Zero-Order Hold12/1
  [TSC] -> Zero-Order Hold13/1
  Zero-Order Hold13/1 -> MATLAB Function3/3(uc)
  Zero-Order Hold12/1 -> MATLAB Function3/2(ub)
  Zero-Order Hold8/1 -> MATLAB Function3/1(ua)
  [IL] -> Zero-Order Hold14/1
  Demux1/3 -> MATLAB Function3/6(ic)
  Zero-Order Hold14/1 -> Demux1/1
  Demux1/2 -> MATLAB Function3/5(ib)
  Demux1/1 -> MATLAB Function3/4(ia)
  MATLAB Function3/1(U1) -> [U1]
  MATLAB Function3/2(V1) -> [V1]
  MATLAB Function3/3(W1) -> [W1]
  MATLAB Function3/4(U2) -> [U2]
  MATLAB Function3/5(V2) -> [V2]
  MATLAB Function3/6(W2) -> [W2]
  connections:
  Voltage Measurement/LConn1 -- Three-Phase V-I Measurement3/LConn1 -- Series RLC Branch22/RConn1
  Series RLC Branch18/RConn1 -- Series RLC Branch19/RConn1 -- Series RLC Branch17/RConn1 -- Ground2/LConn1
  Series RLC Branch2/RConn1 -- Series RLC Branch27/LConn1 -- Series RLC Branch4/LConn1
  Series RLC Branch27/RConn1 -- Series RLC Branch25/RConn1 -- Series RLC Branch26/RConn1
  Series RLC Branch15/RConn1 -- Series RLC Branch25/LConn1 -- Series RLC Branch22/LConn1
  Series RLC Branch1/RConn1 -- Series RLC Branch26/LConn1 -- Series RLC Branch3/LConn1
  Series RLC Branch3/RConn1 -- Voltage Measurement/LConn2 -- Three-Phase V-I Measurement3/LConn2
  Series RLC Branch15/LConn1 -- Three-Phase V-I Measurement2/RConn1
  Series RLC Branch2/LConn1 -- Three-Phase V-I Measurement2/RConn3
  Series RLC Branch1/LConn1 -- Three-Phase V-I Measurement2/RConn2
  Voltage Measurement2/LConn1 -- Mosfet6/LConn1 -- Mosfet8/LConn1 -- Mosfet10/LConn1 -- Series RLC Branch14/LConn1 -- DC Voltage Source1/RConn1
  Mosfet5/RConn1 -- Mosfet11/LConn1 -- Three-Phase V-I Measurement2/LConn3 -- Mosfet10/RConn1
  Series RLC Branch14/RConn1 -- Voltage Measurement2/LConn2 -- Series RLC Branch16/LConn1 -- Voltage Measurement4/LConn1 -- Mosfet4/RConn1 -- Mosfet/RConn1 -- Mosfet2/RConn1
  Mosfet3/RConn1 -- Three-Phase V-I Measurement2/LConn2 -- Mosfet9/LConn1 -- Mosfet8/RConn1
  Mosfet6/RConn1 -- Three-Phase V-I Measurement2/LConn1 -- Mosfet7/LConn1 -- Mosfet1/RConn1
  Voltage Measurement4/LConn2 -- Series RLC Branch16/RConn1 -- Mosfet7/RConn1 -- Mosfet11/RConn1 -- Mosfet9/RConn1 -- DC Voltage Source1/LConn1
  Mosfet2/LConn1 -- Mosfet3/LConn1
  Mosfet4/LConn1 -- Mosfet5/LConn1
  Mosfet/LConn1 -- Mosfet1/LConn1
  Series RLC Branch4/RConn1 -- Three-Phase V-I Measurement3/LConn3
  Three-Phase V-I Measurement3/RConn3 -- Series RLC Branch19/LConn1
  Series RLC Branch18/LConn1 -- Three-Phase V-I Measurement3/RConn2
  Three-Phase V-I Measurement3/RConn1 -- Series RLC Branch17/LConn1

== matlab function ThreeLevel_Ttype_OffGrid_Inverter_Sim/MATLAB Function1 ==
  data: d input; a output; q input; theta input; b output; c output
function [a, b, c] = dq_to_abc_90deg(d, q, theta)
% ######################################################################
% 2输入 (d, q) -> 3输出 (a, b, c) 的分立式同步旋转坐标反变换
% 严格匹配 Simulink 模式: dq0 to abc (90 degrees behind phase A axis)
% ######################################################################

    % ----------- 1. 三角函数预计算 -----------
    cos_theta = cos(theta);
    sin_theta = sin(theta);

    % ----------- 2. 修正后的反帕克变换 (dq -> alpha/beta) -----------
    % 严格匹配 90 degrees behind 模式的数学逆运算
    alpha = d * sin_theta + q * cos_theta;
    beta  = -d * cos_theta + q * sin_theta;

    % ----------- 3. 标准等幅值反克拉克变换 (alpha/beta -> abc) -----------
    k2 = 1.0 / 2.0;
    k3 = sqrt(3.0) / 2.0;
    
    a = alpha;
    b = -k2 * alpha + k3 * beta;
    c = -k2 * alpha - k3 * beta;

end

== matlab function ThreeLevel_Ttype_OffGrid_Inverter_Sim/MATLAB Function3 ==
  data: ua input; U1 output; ub input; uc input; ia input; ib input; ic input; V1 output; W1 output; U2 output; V2 output; W2 output; uo output
function [U1, V1, W1, U2, V2, W2, uo] = calc_zero_sequence_voltage_six_outputs(ua, ub, uc, ia, ib, ic)
% #codegen
% =========================================================================
% 功能: 物理量纲对齐版零序电压注入法（彻底消除高频震荡与波形畸变）
% 适用架构: 针对 T 型三电平（T-Type 3-Level）逆变器，配合 PD-PWM 深度优化
% 
% 输入参数：
%   ua, ub, uc  - 三相归一化电压基准信号 (范围通常在 -1.0 到 1.0 之间)
%   ia, ib, ic  - 三相实际反馈电流采样值 (单位：A)
% 
% 输出参数：
%   U1, V1, W1  - 用于配置硬件第一组比较寄存器的 PWM 计数器值 (对应正负半周切换)
%   U2, V2, W2  - 用于配置硬件第二组比较寄存器的 PWM 计数器值 (带 ARR 偏置)
%   uo          - 最终计算并输出的零序注入电压值 (Zero-Sequence Voltage)
% =========================================================================

    % ARR (Auto-Reload Register): 定时器自动重装载值
    % 用于将标幺化调制波 [-1, 1] 映射到数字硬件实际的寄存器计数周期
    ARR = 8500.0;
    
    % === 核心安全与稳定性控制参数 ===
    HYSTERESIS = 0.03;        % 扇区切换滞环宽度：防止三相电压在过零点附近微小抖动导致扇区频繁跳变
    EPSILON = 0.05;           % 奇异点防御下限：当电流分母接近零时，用于限幅，防止计算出的零序电压飞走
    SMOOTHING_FACTOR = 0.3;   % 一阶低通滤波器系数：值越小滤波越强，用以平滑零序电压的高频纹波
    
    % === 状态持久化变量（用于滞环控制和一阶滤波） ===
    persistent sa_prev sb_prev sc_prev uo_prev
    if isempty(sa_prev)
        sa_prev = 1;          % A相上一次的电压符号状态 (1: 正半周, -1: 负半周)
        sb_prev = 1;          % B相上一次的电压符号状态
        sc_prev = 1;          % C相上一次的电压符号状态
        uo_prev = 0;          % 上一次迭代最终输出的零序电压
    end
    
    %% 1. 带滞环的三相电压符号/半周判断
    % 目的：确定当前空间电压矢量所处的扇区。利用滞环消除采样噪声带来的瞬时误判。
    sa = sign_with_hysteresis(ua, HYSTERESIS, sa_prev);
    sb = sign_with_hysteresis(ub, HYSTERESIS, sb_prev);
    sc = sign_with_hysteresis(uc, HYSTERESIS, sc_prev);
    
    % 更新历史状态，供下一次控制周期使用
    sa_prev = sa;
    sb_prev = sb;
    sc_prev = sc;
    
    %% 2. 纯前馈中点瞬时平衡计算 (NP Balance Feedforward)
    % 物理原理：三电平逆变器在小矢量阶段会抽头连接到直流侧中点（NP）。
    % 根据当前三相开关管的导通组合，中点电流 i_NP 可由三相电流组合表达。
    % 通过注入零序电压 uo_forward，动态改变各相中点动作时间，使瞬时中点电流积分为 0。
    % 公式推导自：u_forward = P_mid / I_mid_sum
    if (sa > 0) && (sb < 0) && (sc < 0)
        num = -ua*ia + ub*ib + uc*ic;
        den = ia - ib - ic;
    elseif (sa > 0) && (sb > 0) && (sc < 0)
        num = -ua*ia - ub*ib + uc*ic;
        den = ia + ib - ic;
    elseif (sa < 0) && (sb > 0) && (sc < 0)
        num = ua*ia - ub*ib + uc*ic;
        den = -ia + ib - ic;
    elseif (sa < 0) && (sb > 0) && (sc > 0)
        num = ua*ia - ub*ib - uc*ic;
        den = -ia + ib + ic;
    elseif (sa < 0) && (sb < 0) && (sc > 0)
        num = ua*ia + ub*ib + uc*ic;
        den = -ia - ib + ic;
    elseif (sa > 0) && (sb < 0) && (sc > 0)
        num = -ua*ia + ub*ib - uc*ic;
        den = ia - ib + ic;
    else
        % 理论上三相平衡时不会进入此区间（如 sa=sb=sc 均为正或均为负，不符合SPWM调制逻辑）
        num = 0;
        den = 1;
    end
    
    %% 3. 分母死区与奇异点安全处理
    % 物理风险：当分母（合成中点电流能力值）无限接近于 0 时（如电机空载或电流过零点），
    % 直接相除会导致 uo_forward 爆炸，引起系统高频共振。
    if abs(den) < EPSILON
        % 强行将分母限幅在最小安全阈值 EPSILON，同时保持其原本的正负号
        den_safe = EPSILON * sign(den);
        if den_safe == 0, den_safe = EPSILON; end % 防御 sign(0) = 0 的情况
        uo_forward = num / den_safe;
    else
        uo_forward = num / den;
    end
    
    %% 4. 原始零序电压计算
    % 纯前馈控制模式：仅通过瞬时电流和电压计算所需的零序注入量
    % 负责消灭由负载电流不对称带来的3倍频中点电压波动
    uo_raw = uo_forward;
    
    %% 5. 调制波边界动态限幅与符号安全防御
    % 5.1 线性调制区硬限幅
    % 注入零序电压后，绝对不能让最终的三相调制波（u + uo）超出 [-1, 1] 的物理边界
    uo_max =  1.0 - max([ua, ub, uc]); % 能够向上抬升的最大空间
    uo_min = -1.0 - min([ua, ub, uc]); % 能够向下压低的最小空间
    uo_local = max(min(uo_raw, uo_max), uo_min);
    
    % 5.2 符号防御机制 (Phase-Reversal Protection)
    % 物理风险：如果注入的零序电压太大，导致原本处于正半周的调制波（ua+uo）变成了负值，
    % 或者原本处于负半周的变成了正值，会导致 T 型拓扑的开关管瞬时误导通，引发严重的波形畸变。
    % 逻辑判断：一旦发现任何一相的物理符号在注入后发生翻转，立即放弃当前的激进注入，退守至上一次安全值的 50%。
    if (sa > 0 && (ua + uo_local) <= 0) || (sa < 0 && (ua + uo_local) >= 0) || ...
       (sb > 0 && (ub + uo_local) <= 0) || (sb < 0 && (ub + uo_local) >= 0) || ...
       (sc > 0 && (uc + uo_local) <= 0) || (sc < 0 && (uc + uo_local) >= 0)
        uo_local = 0.5 * uo_prev;
    end
    
    %% 6. 一阶低通动态滤波 (Smoothing Filter)
    % 目的：消除由于电流/电压离散采样带来的尖峰噪声，使注入的零序电压波形平滑连续。
    uo_filtered = SMOOTHING_FACTOR * uo_local + (1 - SMOOTHING_FACTOR) * uo_prev;
    uo_prev = uo_filtered;  % 记忆当前滤波值，供下一周期使用
    uo = uo_filtered;       % 最终输出的零序电压
    
    %% 7. 最终调制波生成与硬件定时器量化量转换
    % 7.1 将零序电压注入到原始调制波中，并对边界进行 [-1, 1] 的终极闭锁限制
    sa_norm = clamp(ua + uo, -1, 1);
    sb_norm = clamp(ub + uo, -1, 1);
    sc_norm = clamp(uc + uo, -1, 1);
    
    % 7.2 物理量映射到硬件定时器寄存器值
    % 针对 PD-PWM (Phase Disposition PWM) 的两组载波配置：
    % 第一组比较值（U1, V1, W1）：处理正半周调制，范围映射到 [0, ARR] （当 *_norm 从 -1 到 1）
    U1 = sa_norm * ARR;
    V1 = sb_norm * ARR;
    W1 = sc_norm * ARR;
    
    % 第二组比较值（U2, V2, W2）：处理负半周载波的基准对齐，整体往上平移一个完整的 ARR 周期
    U2 = U1 + ARR;
    V2 = V1 + ARR;
    W2 = W1 + ARR;
end

%% ========================== 辅助子函数 ==========================

function s = sign_with_hysteresis(x, h, x_prev)
% 功能：带滞环的符号提取函数
% 参数：x - 当前输入值, h - 滞环半宽, x_prev - 上一次的符号状态
% 逻辑：只有当输入超出滞环阈值时才切换状态，在中心死区内保持历史状态，可有效抑制零点噪声。
    if x > h
        s = 1;
    elseif x < -h
        s = -1;
    else
        s = x_prev; % 落在死区内，维持现状
    end
end

function y = clamp(x, min_val, max_val)
% 功能：标准的数值限幅截断函数
    y = max(min(x, max_val), min_val);
end

== matlab function ThreeLevel_Ttype_OffGrid_Inverter_Sim/MATLAB Function2 ==
  data: Ua_norm input; U1 output; Ub_norm input; V1 output; W1 output; U2 output; V2 output; W2 output; Uc_norm input
function [U1, V1, W1, U2, V2, W2] = svpwm_3level_paper_verify(Ua_norm, Ub_norm, Uc_norm)
% #codegen
% =========================================================================
% 功能: 结构优化版三电平NPC逆变器SVPWM算法（内置输入归一化与克拉克变换）
% =========================================================================

%% 0. 系统常数定义与输入反归一化
Udc   = 60;              % 固定的直流母线电压 (V)
ARR   = 8500;            % 半个开关周期计数值（完整周期2*ARR）
sqrt3 = 1.732050807568877;
inv_sqrt3 = 0.577350269189626; % 1/sqrt(3)

% 将归一化的 [-1, 1] 输入还原为实际的物理电压基准值
V_base = Udc * inv_sqrt3; 
Va = Ua_norm * V_base;
Vb = Ub_norm * V_base;
Vc = Uc_norm * V_base;

%% 1. 内置克拉克变换 (abc -> alpha/beta)
Valpha = (2.0 / 3.0) * Va - (1.0 / 3.0) * Vb - (1.0 / 3.0) * Vc;
Vbeta  = inv_sqrt3 * Vb - inv_sqrt3 * Vc;

%% ================== 第一步：大扇区判断 (N因子法) ==================
A = Vbeta;
B = (sqrt3/2) * Valpha - 0.5 * Vbeta;
C = -(sqrt3/2) * Valpha - 0.5 * Vbeta;
a = double(A > 0);
b = double(B > 0);
c = double(C > 0);
N = a + 2*b + 4*c;

% 【安全卡口】当输入全为0导致 N=0 时，强制令 N=3（对应 sector_map(3) = 1 扇区）防止仿真死机
if N == 0
    N = 3; 
end

sector_map = [2, 6, 1, 4, 3, 5]; 
S_big = sector_map(N);

%% ================== 第二步：小扇区判断 (空间旋转与直线方程) ==================
theta_global = atan2(Vbeta, Valpha);
if theta_global < 0
    theta_global = theta_global + 2*pi;
end
% 空间对称旋转，收敛至第一大扇区 [0, pi/3]
theta1 = theta_global - double(S_big - 1) * (pi/3);
Vamp = sqrt(Valpha^2 + Vbeta^2);
Valpha1 = Vamp * cos(theta1);
Vbeta1 = Vamp * sin(theta1);

% 执行二叉决策树判定小扇区
if theta1 >= pi/6
    if (Vbeta1 - (sqrt3/6)*Udc) >= 0
        S_small = 6; 
    else
        if (-sqrt3*Valpha1 - Vbeta1 + (sqrt3/3)*Udc) >= 0
            S_small = 2; 
        else
            S_small = 4; 
        end
    end
else
    if (sqrt3*Valpha1 - Vbeta1 - (sqrt3/3)*Udc) >= 0
        S_small = 5; 
    else
        if (-sqrt3*Valpha1 - Vbeta1 + (sqrt3/3)*Udc) >= 0
            S_small = 1; 
        else
            S_small = 3; 
        end
    end
end

%% ================== 第三步：合成矢量时间计算 ==================
m = (sqrt3 * Vamp) / Udc;
m = min(m, 1.1547); % 三电平SVPWM最大线性调制比
Ta = 0; Tb = 0; Tc = 0;
switch S_small
    case {1, 2} 
        Ta = 2 * m * ARR * sin(theta1);
        Tb = ARR - 2 * m * ARR * sin(pi/3 + theta1);
        Tc = 2 * m * ARR * sin(pi/3 - theta1);
        
    case {3, 4} 
        Ta = ARR - 2 * m * ARR * sin(theta1);
        Tb = -ARR + 2 * m * ARR * sin(pi/3 + theta1);
        Tc = ARR - 2 * m * ARR * sin(pi/3 - theta1);
        
    case 5 
        Ta = 2 * m * ARR * sin(theta1);
        Tb = 2 * ARR - 2 * m * ARR * sin(pi/3 + theta1);
        Tc = -ARR + 2 * m * ARR * sin(pi/3 - theta1);
        
    case 6 
        Ta = -ARR + 2 * m * ARR * sin(theta1);
        Tb = 2 * ARR - 2 * m * ARR * sin(pi/3 + theta1);
        Tc = 2 * m * ARR * sin(pi/3 - theta1);
end

%% ================== 第四步：工程过调制保护与限幅 ==================
if Ta < 0, Ta = 0; end
if Tb < 0, Tb = 0; end
if Tc < 0, Tc = 0; end
Tsum = Ta + Tb + Tc;
if Tsum > ARR
    scale = ARR / Tsum;
    Ta = Ta * scale;
    Tb = Tb * scale;
    Tc = Tc * scale;
end

%% ================== 第五步：直观的基础调制分量计算 ==================
m_high = 0; m_mid = 0; m_low = 0;
if mod(S_big, 2) ~= 0
    % ----------------- 奇数大扇区时的时间分配 -----------------
    switch S_small
        case 1
            m_high = (Tc/2) / ARR;
            m_mid  = (-Tc/2) / ARR;
            m_low  = (-Tc/2 - Ta) / ARR;
        case 2
            m_high = (Tc + Ta/2) / ARR;
            m_mid  = (Ta/2) / ARR;
            m_low  = (-Ta/2) / ARR;
        case 3
            m_high = (Tb + Ta/2) / ARR;
            m_mid  = (-Ta/2) / ARR;
            m_low  = -(ARR - Ta/2) / ARR;
        case 4
            m_high = (ARR - Tc/2) / ARR;
            m_mid  = (Tc/2) / ARR;
            m_low  = (-Tc/2 - Tb) / ARR;
        case 5
            m_high = (ARR - Tb/2) / ARR;
            m_mid  = (-Tb/2 - Tc) / ARR;  
            m_low  = -(ARR - Tb/2) / ARR;
        case 6
            m_high = (ARR - Tb/2) / ARR;
            m_mid  = (Ta + Tb/2) / ARR;
            m_low  = -(ARR - Tb/2) / ARR;
    end
else
    % ----------------- 偶数大扇区时的时间分配 -----------------
    switch S_small
        case 1
            m_high = (Ta + Tc/2) / ARR;    
            m_mid  = (Tc/2) / ARR;         
            m_low  = (-Tc/2) / ARR;        
        case 2
            m_high = (Ta/2) / ARR;
            m_mid  = (-Ta/2) / ARR;
            m_low  = (-Ta/2 - Tc) / ARR;
        case 3
            m_high = (ARR - Ta/2) / ARR;
            m_mid  = (Ta/2) / ARR;
            m_low  = (-Ta/2 - Tb) / ARR;  
        case 4
            m_high = (Tb + Tc/2) / ARR;
            m_mid  = (-Tc/2) / ARR;
            m_low  = -(ARR - Tc/2) / ARR;
        case 5
            m_high = (ARR - Tb/2) / ARR;
            m_mid  = (Tc + Tb/2) / ARR;
            m_low  = -(ARR - Tb/2) / ARR;
        case 6
            m_high = (ARR - Tb/2) / ARR;
            m_mid  = (-Ta - Tb/2) / ARR;
            m_low  = -(ARR - Tb/2) / ARR;
    end
end

%% ================== 第六步：物理三相直接映射 (归一化 [-1,1]) ==================
U_norm = 0; V_norm = 0; W_norm = 0;
switch S_big
    case 1  % 大扇区1: A > B > C
        U_norm = m_high;  V_norm = m_mid;   W_norm = m_low;
    case 2  % 大扇区2: B > A > C
        U_norm = m_mid;   V_norm = m_high;  W_norm = m_low;
    case 3  % 大扇区3: B > C > A
        U_norm = m_low;   V_norm = m_high;  W_norm = m_mid;
    case 4  % 大扇区4: C > B > A
        U_norm = m_low;   V_norm = m_mid;   W_norm = m_high;
    case 5  % 大扇区5: C > A > B
        U_norm = m_mid;   V_norm = m_low;   W_norm = m_high;
    case 6  % 大扇区6: A > C > B
        U_norm = m_high;  V_norm = m_low;   W_norm = m_mid;
end

%% ================== 第七步：硬件计数域缩放与双波复制 ==================
% 1. 第一组调制波：直接放大到定时器半周期计数值域 [-8500, 8500]
U1 = U_norm * double(ARR);
V1 = V_norm * double(ARR);
W1 = W_norm * double(ARR);

% 2. 第二组调制波：在第一组的基础上整体向上抬升一个 ARR，范围变为 [0, 17000]
U2 = U1 + double(ARR);
V2 = V1 + double(ARR);
W2 = W1 + double(ARR);

end

== matlab function ThreeLevel_Ttype_OffGrid_Inverter_Sim/生成20khz的θ ==
  data: theta output
function theta = gen_theta()
% 无输入，输出 θ (0~2π)
% 控制频率 20kHz，输出基波 50Hz

persistent theta_val step_theta;

if isempty(theta_val)
    % 初始化
    theta_val = 0;          % 初始相位
    f = 50;                 % 输出频率 50Hz
    fs = 20000;             % 控制频率 20kHz
    step_theta = 2*pi*f/fs; % 每步相位增量
end

% 相位累加
theta_val = theta_val + step_theta;

% 相位限幅 0 ~ 2π
if theta_val >= 2*pi
    theta_val = theta_val - 2*pi;
end

% 输出
theta = theta_val;
end

== matlab function ThreeLevel_Ttype_OffGrid_Inverter_Sim/adc转dq3 ==
  data: a input; b input; c input; d output; theta input; q output
function [d, q] = abc_to_dq_90deg(a, b, c, theta)
% ######################################################################
% 3输入 (a, b, c, theta) -> 2输出 (d, q) 的分立式坐标变换
% 严格匹配 Simulink 模式: 90 degrees behind phase A axis
% ######################################################################

    % ----------- 1. 分立式克拉克变换 (abc -> alpha/beta) -----------
    % 采用等幅值标准系数
    alpha = (2.0 / 3.0) * a - (1.0 / 3.0) * b - (1.0 / 3.0) * c;
    beta  = (1.0 / sqrt(3.0)) * b - (1.0 / sqrt(3.0)) * c;

    % ----------- 2. 三角函数计算 -----------
    cos_theta = cos(theta);
    sin_theta = sin(theta);

    % ----------- 3. 修正后的帕克变换 (匹配 90 deg behind 逻辑) -----------
    % 注意：这里的正负号和三角函数组合与 0 度对齐不同
    d =  alpha * sin_theta - beta * cos_theta;
    q =  alpha * cos_theta + beta * sin_theta;

end

== matlab function ThreeLevel_Ttype_OffGrid_Inverter_Sim/adc转dq1 ==
  data: a input; b input; c input; d output; theta input; q output
function [d, q] = abc_to_dq_90deg(a, b, c, theta)
% ######################################################################
% 3输入 (a, b, c, theta) -> 2输出 (d, q) 的分立式坐标变换
% 严格匹配 Simulink 模式: 90 degrees behind phase A axis
% ######################################################################

    % ----------- 1. 分立式克拉克变换 (abc -> alpha/beta) -----------
    % 采用等幅值标准系数
    alpha = (2.0 / 3.0) * a - (1.0 / 3.0) * b - (1.0 / 3.0) * c;
    beta  = (1.0 / sqrt(3.0)) * b - (1.0 / sqrt(3.0)) * c;

    % ----------- 2. 三角函数计算 -----------
    cos_theta = cos(theta);
    sin_theta = sin(theta);

    % ----------- 3. 修正后的帕克变换 (匹配 90 deg behind 逻辑) -----------
    % 注意：这里的正负号和三角函数组合与 0 度对齐不同
    d =  alpha * sin_theta - beta * cos_theta;
    q =  alpha * cos_theta + beta * sin_theta;

end
